simulink model "simulink_PD"  (R2024b)
settings: Solver=ode4  StartTime=0.0  StopTime=20  FixedStep=1e-3  RelTol=1e-3  EnableMultiTasking=on
values from neighbouring files (symbols this model uses):
  Kd = 100    [MAIN.m]
  Kp = 20000    [MAIN.m]
  noise = 0    [MAIN.m]
  V_ref = 60/3.6    (= 16.6666666667)    [MAIN.m]
undefined symbols (not defined in the file or in its folder): par
libraries: simulink x2
settings Model: Creator=bshyrokau  LastModifiedBy=nicvi
settings SolverCC: AlgebraicLoopSolver=TrustRegion
settings DataIOCC: SaveOutput=off  SignalLogging=off  DSMLogging=off  SaveTime=off  ReturnWorkspaceOutputs=off
settings OptimizationCC: ReuseModelBlockBuffer=off  LifeSpan=inf
settings DebuggingCC: UnconnectedInputMsg=warning  UnconnectedOutputMsg=warning  UnconnectedLineMsg=warning  AllowSymbolicDim=off  SFUnexpectedBacktrackingDiag=warning  SFNoUnconditionalDefaultTransitionDiag=warning  SFExecutionAtInitializationDiag=none  ArithmeticOperatorsInVariantConditions=warning
settings ModelReferenceCC: EnableRefExpFcnMdlSchedulingChecks=on  PropagateSignalLabelsOutOfModel=off
settings SFSimCC: SimUseLocalCustomCode=off  CustomCodeUndefinedFunction=UseInterfaceOnly
settings RTWCC: RTWUseLocalCustomCode=off  GPUComputeCapability=3.5  DLArmComputeVersion=19.05
settings CodeAppCC: StateflowObjectComments=on
settings GRTTargetCC: TargetLangStandard=C89/C90 (ANSI)
settings ConfigComp: CovMetricSettings=dw  CovSaveCumulativeToWorkspaceVar=on  CovSaveSingleToWorkspaceVar=on  CovExternalEMLEnable=off
settings SimscapeCC: SimscapeNormalizeSystem=off
settings ConfigurationSet: Description=SimMechanics 2G

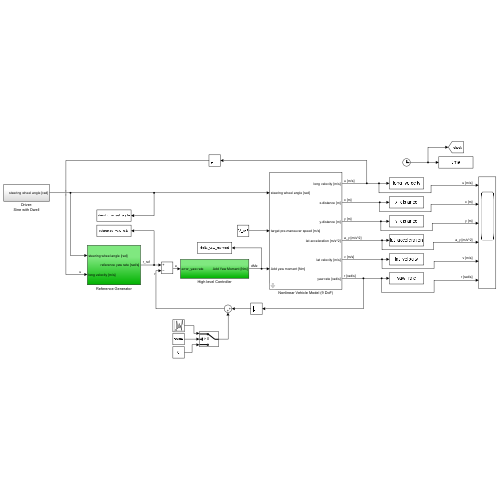
[thumbnail: Simulink's stored preview of the top-level diagram]
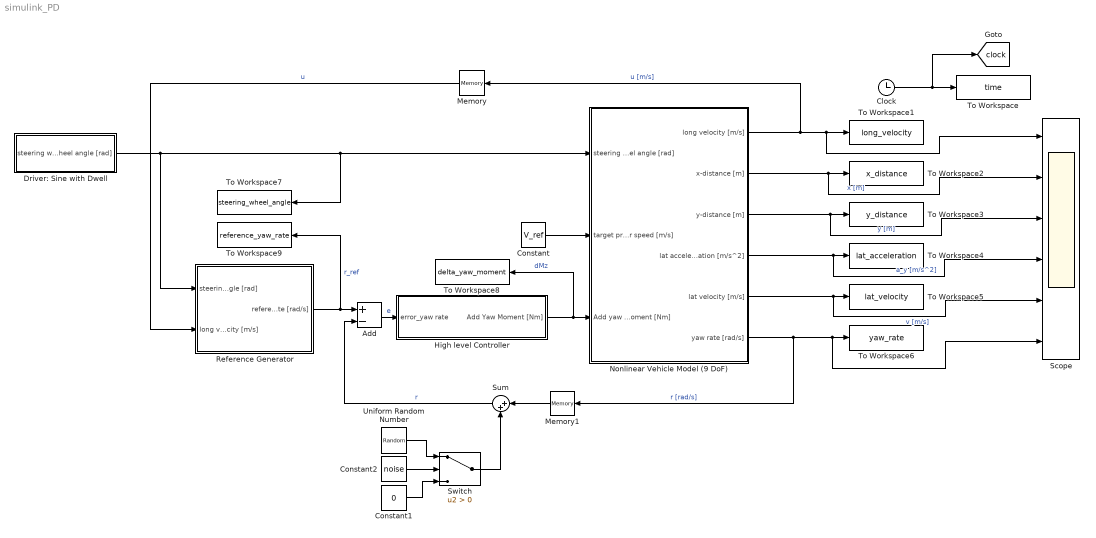
== system simulink_PD ==
  Add : Sum  Inputs=+-
  Clock : Clock
  Constant : Constant  Value=V_ref
  Constant1 : Constant  Value=0
  Constant2 : Constant  Value=noise
  Driver: Sine with Dwell : Subsystem
  High level Controller : Subsystem
  Memory : Memory
  Memory1 : Memory
  Nonlinear Vehicle Model (9 DoF) : Subsystem
      mask help: Simulink:masks:GenSFuncDesc_MD
      mask Help: eval('feval(''rtwprivate'',''rtwhelpview'',''rtw_sfcn_block'')');
  Reference Generator : Subsystem
  Scope : Scope  NumInputPorts=6
  Sum : Sum  Inputs=|++
  Switch : Switch  Criteria=u2 > Threshold  SaturateOnIntegerOverflow=off  InputSameDT=off
  To Workspace : ToWorkspace  VariableName=time  SampleTime=-1
  To Workspace1 : ToWorkspace  VariableName=long_velocity  SampleTime=-1
  To Workspace2 : ToWorkspace  VariableName=x_distance  SampleTime=-1
  To Workspace3 : ToWorkspace  VariableName=y_distance  SampleTime=-1
  To Workspace4 : ToWorkspace  VariableName=lat_acceleration  SampleTime=-1
  To Workspace5 : ToWorkspace  VariableName=lat_velocity  SampleTime=-1
  To Workspace6 : ToWorkspace  VariableName=yaw_rate  SampleTime=-1
  To Workspace7 : ToWorkspace  VariableName=steering_wheel_angle  SampleTime=-1
  To Workspace8 : ToWorkspace  VariableName=delta_yaw_moment  SampleTime=-1
  To Workspace9 : ToWorkspace  VariableName=reference_yaw_rate  SampleTime=-1
  Uniform Random Number : UniformRandomNumber  Minimum=-deg2rad(0.5)  Maximum=deg2rad(0.5)  SampleTime=0.001
  tag scope: clock=global
  wires:
  Driver: Sine with Dwell/1(steering wheel angle [rad]) -> Nonlinear Vehicle Model (9 DoF)/1(steering wheel angle [rad]), To Workspace7/1, Reference Generator/1(steering wheel angle [rad])
  Reference Generator/1(reference yaw rate [rad/s]) -> To Workspace9/1, Add/1  "r_ref"
  High level Controller/1(Add Yaw Moment [Nm]) -> To Workspace8/1, Nonlinear Vehicle Model (9 DoF)/3(Add yaw moment [Nm])  "dMz"
  Add/1 -> High level Controller/1(error_yaw rate)  "e"
  Nonlinear Vehicle Model (9 DoF)/6(yaw rate [rad/s]) -> Scope/6, To Workspace6/1, Memory1/1  "r [rad/s]"
  Nonlinear Vehicle Model (9 DoF)/5(lat velocity [m/s]) -> Scope/5, To Workspace5/1  "v [m/s]"
  Nonlinear Vehicle Model (9 DoF)/1(long velocity [m/s]) -> Scope/1, To Workspace1/1, Memory/1  "u [m/s]"
  Nonlinear Vehicle Model (9 DoF)/4(lat acceleration [m/s^2]) -> Scope/4, To Workspace4/1  "a_y [m/s^2]"
  Nonlinear Vehicle Model (9 DoF)/2(x-distance [m]) -> Scope/2, To Workspace2/1  "x [m]"
  Nonlinear Vehicle Model (9 DoF)/3(y-distance [m]) -> Scope/3, To Workspace3/1  "y [m]"
  Constant/1 -> Nonlinear Vehicle Model (9 DoF)/2(target pre-maneuver speed [m/s])
  Clock/1 -> [clock], To Workspace/1
  Memory/1 -> Reference Generator/2(long velocity [m/s])  "u"
  Memory1/1 -> Sum/1
  Uniform Random Number/1 -> Switch/1
  Sum/1 -> Add/2  "r"
  Switch/1 -> Sum/2
  Constant1/1 -> Switch/3
  Constant2/1 -> Switch/2

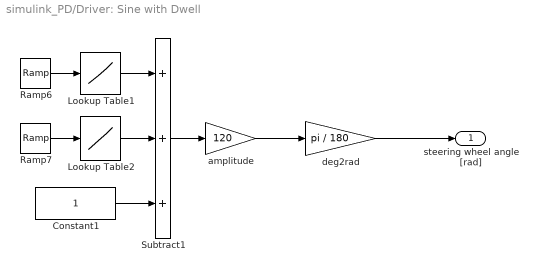
== system simulink_PD/Driver: Sine with Dwell ==
  Constant1 : Constant
  Lookup Table1 : Lookup  InputValues=[0:0.1:3*pi/2 3*pi/2+eps]*0.7  Table=sin([0:0.1:3*pi/2 3*pi/2+eps])  LookUpMeth=Interpolation-Use End Values  SaturateOnIntegerOverflow=off
  Lookup Table2 : Lookup  InputValues=[3*pi/2:0.1:2*pi 2*pi+eps]*0.7  Table=sin([3*pi/2:0.1:2*pi 2*pi+eps])  LookUpMeth=Interpolation-Use End Values  SaturateOnIntegerOverflow=off
  Ramp6 : simulink/Sources/Ramp  slope=pi  start=10  InitialOutput=0
  Ramp7 : simulink/Sources/Ramp  slope=pi  start=10+0.5  InitialOutput=0
  Subtract1 : Sum  Inputs=+++
  amplitude : Gain  Gain=120
  deg2rad : Gain  Gain=pi / 180
  steering wheel angle [rad] : Outport  VectorParamsAs1DForOutWhenUnconnected=off
  wires:
  Ramp6/1 -> Lookup Table1/1
  Ramp7/1 -> Lookup Table2/1
  Lookup Table2/1 -> Subtract1/2
  Lookup Table1/1 -> Subtract1/1
  Constant1/1 -> Subtract1/3
  Subtract1/1 -> amplitude/1
  amplitude/1 -> deg2rad/1
  deg2rad/1 -> steering wheel angle [rad]/1

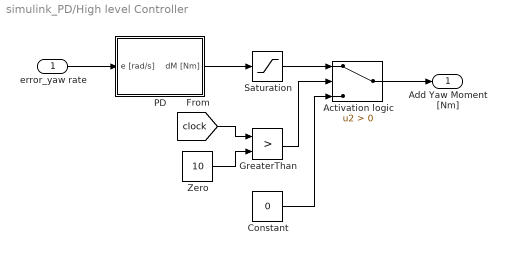
== system simulink_PD/High level Controller ==
  error_yaw rate : Inport
  Activation logic : Switch  Criteria=u2 > Threshold  SaturateOnIntegerOverflow=off  InputSameDT=off
  Constant : Constant  Value=0
  GreaterThan : RelationalOperator  Operator=>  OutDataTypeStr=boolean  RndMeth=Simplest  InputSameDT=off
  PD : Subsystem
  Saturation : Saturate  UpperLimit=10000  LowerLimit=-10000
  Zero : Constant  Value=10  OutDataTypeStr=Inherit: Inherit via back propagation
  Add Yaw Moment [Nm] : Outport  VectorParamsAs1DForOutWhenUnconnected=off
  wires:
  error_yaw rate/1 -> PD/1(e [rad/s])
  Saturation/1 -> Activation logic/1
  PD/1(dM [Nm]) -> Saturation/1
  Activation logic/1 -> Add Yaw Moment [Nm]/1
  Constant/1 -> Activation logic/3
  Zero/1 -> GreaterThan/2
  [clock] -> GreaterThan/1
  GreaterThan/1 -> Activation logic/2

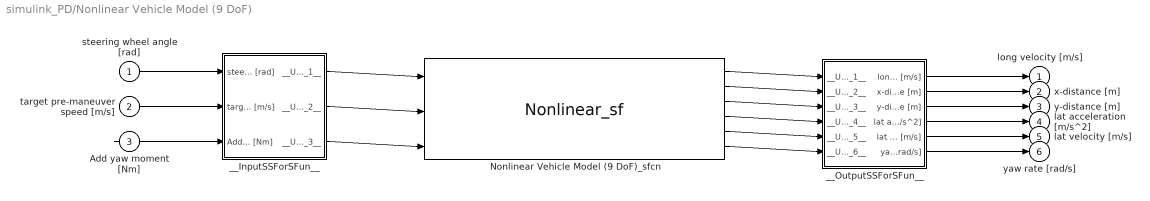
== system simulink_PD/Nonlinear Vehicle Model (9 DoF) ==
  steering wheel angle [rad] : Inport
  target pre-maneuver speed [m/s] : Inport  Port=2
  Add yaw moment [Nm] : Inport  Port=3
  Nonlinear Vehicle Model (9 DoF)_sfcn : S-Function  FunctionName=Nonlinear_sf  SFunctionModules=""  SFunctionDeploymentMode=off  EnableBusSupport=off  mask{rtw_sf_name=Nonlinear_sf, showVar=off}
      mask prompts: rtw_sf_name "Simulink:masks:GenSFuncName_MP"; showVar "Simulink:masks:GenSFuncShowModuleList_MP"
      mask help: Simulink:masks:GenSFuncDesc_MD
      mask init:
      | displist = '';
      | if ~strcmp(get_param(gcb, 'FunctionName'), rtw_sf_name);
      |   set_param(gcb, 'FunctionName', rtw_sf_name);
      | end
      | % Check if we are generating code
      | rtw_mode = false;
      | if strcmpi(get_param(bdroot(gcb),'SimulationStatus'),'Initializing')
      | 	rtw_mode = strcmpi(get_param(bdroot(gcb),'BuildingRTWCode'),'on') && ...
      | 		~strcmpi(get_param(bdroot(gcb),'TargetStyle'),'SimulationTarget');
      | end
      | if showVar || rtw_mode
      | 	if exist('rtwsfunc') == 2 | exist('rtwsfunc') == 6
      | 		tmplist = rtwsfunc(rtw_sf_name,gcb);
      | 		tmplist = DAStudio.message('Simulink:masks:GenSFuncListOfModules_IC', tmplist);
      | 	elseif showVar
      | 		tmplist1 = DAStudio.message('Simulink:masks:GenSFuncListOfModules_IC', '');
      |         tmplist2 = DAStudio.message('Simulink:masks:GenSFuncNotLicensed_IC');
      |         tmplist = [tmplist1 tmplist2];
      |  	end
      | end
      | if showVar
      |   displist = tmplist;
      | end
      settings: CopyFcn=|
      | if ~strcmp(get_param(gcb,'Linkstatus'),'none') && ...
      | ~strcmp(get_param(gcb,'Linkstatus'),'implicit')
      |   set_param(gcb,'LinkStatus','none');
      | end
      mask Help: eval('feval(''rtwprivate'',''rtwhelpview'',''rtw_sfcn_block'')');
      mask Display:
      | port_label('input',1,'steering wheel angle [rad]');
      | port_label('input',2,'target pre-maneuver speed [m/s]');
      | port_label('input',3,'Add yaw moment [Nm]');
      | port_label('output',1,'long velocity [m/s]');
      | port_label('output',2,'x-distance [m]');
      | port_label('output',3,'y-distance [m]');
      | port_label('output',4,'lat acceleration [m/s^2]');
      | port_label('output',5,'lat velocity [m/s]');
      | port_label('output',6,'yaw rate [rad/s]');
  __InputSSForSFun__ : Subsystem
  __OutputSSForSFun__ : Subsystem
  long velocity [m/s] : Outport  VectorParamsAs1DForOutWhenUnconnected=off
  x-distance [m] : Outport  Port=2  VectorParamsAs1DForOutWhenUnconnected=off
  y-distance [m] : Outport  Port=3  VectorParamsAs1DForOutWhenUnconnected=off
  lat acceleration [m/s^2] : Outport  Port=4  VectorParamsAs1DForOutWhenUnconnected=off
  lat velocity [m/s] : Outport  Port=5  VectorParamsAs1DForOutWhenUnconnected=off
  yaw rate [rad/s] : Outport  Port=6  VectorParamsAs1DForOutWhenUnconnected=off
  wires:
  steering wheel angle [rad]/1 -> __InputSSForSFun__/1(steering wheel angle [rad])
  target pre-maneuver speed [m/s]/1 -> __InputSSForSFun__/2(target pre-maneuver speed [m/s])
  Add yaw moment [Nm]/1 -> __InputSSForSFun__/3(Add yaw moment [Nm])
  __InputSSForSFun__/1(__UniqueOutportName__1__) -> Nonlinear Vehicle Model (9 DoF)_sfcn/1
  __InputSSForSFun__/2(__UniqueOutportName__2__) -> Nonlinear Vehicle Model (9 DoF)_sfcn/2
  __InputSSForSFun__/3(__UniqueOutportName__3__) -> Nonlinear Vehicle Model (9 DoF)_sfcn/3
  Nonlinear Vehicle Model (9 DoF)_sfcn/1 -> __OutputSSForSFun__/1(__UniqueInportName__1__)
  Nonlinear Vehicle Model (9 DoF)_sfcn/2 -> __OutputSSForSFun__/2(__UniqueInportName__2__)
  Nonlinear Vehicle Model (9 DoF)_sfcn/3 -> __OutputSSForSFun__/3(__UniqueInportName__3__)
  Nonlinear Vehicle Model (9 DoF)_sfcn/4 -> __OutputSSForSFun__/4(__UniqueInportName__4__)
  Nonlinear Vehicle Model (9 DoF)_sfcn/5 -> __OutputSSForSFun__/5(__UniqueInportName__5__)
  Nonlinear Vehicle Model (9 DoF)_sfcn/6 -> __OutputSSForSFun__/6(__UniqueInportName__6__)
  __OutputSSForSFun__/1(long velocity [m/s]) -> long velocity [m/s]/1
  __OutputSSForSFun__/2(x-distance [m]) -> x-distance [m]/1
  __OutputSSForSFun__/3(y-distance [m]) -> y-distance [m]/1
  __OutputSSForSFun__/4(lat acceleration [m/s^2]) -> lat acceleration [m/s^2]/1
  __OutputSSForSFun__/5(lat velocity [m/s]) -> lat velocity [m/s]/1
  __OutputSSForSFun__/6(yaw rate [rad/s]) -> yaw rate [rad/s]/1

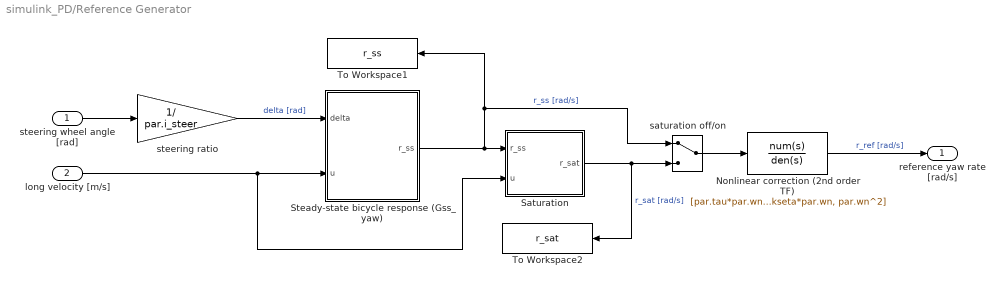
== system simulink_PD/Reference Generator ==
  steering wheel angle [rad] : Inport
  long velocity [m/s] : Inport  Port=2
  Nonlinear correction (2nd order TF) : TransferFcn  Numerator=[par.tau*par.wn^2, par.wn^2]  Denominator=[1, 2*par.kseta*par.wn, par.wn^2]
  Saturation : Subsystem
  Steady-state bicycle response (Gss_yaw) : Subsystem
  To Workspace1 : ToWorkspace  VariableName=r_ss  SampleTime=-1
  To Workspace2 : ToWorkspace  VariableName=r_sat  SampleTime=-1
  saturation off/on : ManualSwitch
  steering ratio : Gain  Gain=1/ par.i_steer
  reference yaw rate [rad/s] : Outport  VectorParamsAs1DForOutWhenUnconnected=off
  wires:
  steering wheel angle [rad]/1 -> steering ratio/1
  steering ratio/1 -> Steady-state bicycle response (Gss_yaw)/1(delta)  "delta [rad]"
  long velocity [m/s]/1 -> Saturation/2(u), Steady-state bicycle response (Gss_yaw)/2(u)
  Steady-state bicycle response (Gss_yaw)/1(r_ss) -> saturation off/on/1, To Workspace1/1, Saturation/1(r_ss)  "r_ss [rad/s]"
  Nonlinear correction (2nd order TF)/1 -> reference yaw rate [rad/s]/1  "r_ref [rad/s]"
  saturation off/on/1 -> Nonlinear correction (2nd order TF)/1
  Saturation/1(r_sat) -> To Workspace2/1, saturation off/on/2  "r_sat [rad/s]"

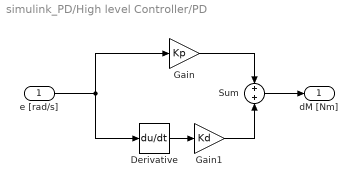
== system simulink_PD/High level Controller/PD ==
  e [rad/s] : Inport
  Derivative : Derivative
  Gain : Gain  Gain=Kp
  Gain1 : Gain  Gain=Kd
  Sum : Sum  Inputs=+|+
  dM [Nm] : Outport
  wires:
  Sum/1 -> dM [Nm]/1
  Gain1/1 -> Sum/2
  Gain/1 -> Sum/1
  e [rad/s]/1 -> Derivative/1, Gain/1
  Derivative/1 -> Gain1/1

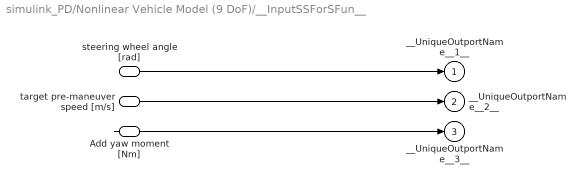
== system simulink_PD/Nonlinear Vehicle Model (9 DoF)/__InputSSForSFun__ ==
  steering wheel angle [rad] : Inport
  target pre-maneuver speed [m/s] : Inport  Port=2
  Add yaw moment [Nm] : Inport  Port=3
  __UniqueOutportName__1__ : Outport
  __UniqueOutportName__2__ : Outport  Port=2
  __UniqueOutportName__3__ : Outport  Port=3
  wires:
  steering wheel angle [rad]/1 -> __UniqueOutportName__1__/1
  target pre-maneuver speed [m/s]/1 -> __UniqueOutportName__2__/1
  Add yaw moment [Nm]/1 -> __UniqueOutportName__3__/1

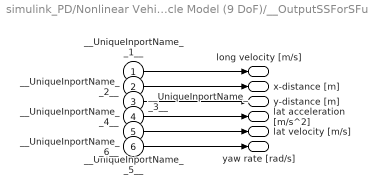
== system simulink_PD/Nonlinear Vehicle Model (9 DoF)/__OutputSSForSFun__ ==
  __UniqueInportName__1__ : Inport
  __UniqueInportName__2__ : Inport  Port=2
  __UniqueInportName__3__ : Inport  Port=3
  __UniqueInportName__4__ : Inport  Port=4
  __UniqueInportName__5__ : Inport  Port=5
  __UniqueInportName__6__ : Inport  Port=6
  long velocity [m/s] : Outport  VectorParamsAs1DForOutWhenUnconnected=off
  x-distance [m] : Outport  Port=2  VectorParamsAs1DForOutWhenUnconnected=off
  y-distance [m] : Outport  Port=3  VectorParamsAs1DForOutWhenUnconnected=off
  lat acceleration [m/s^2] : Outport  Port=4  VectorParamsAs1DForOutWhenUnconnected=off
  lat velocity [m/s] : Outport  Port=5  VectorParamsAs1DForOutWhenUnconnected=off
  yaw rate [rad/s] : Outport  Port=6  VectorParamsAs1DForOutWhenUnconnected=off
  wires:
  __UniqueInportName__1__/1 -> long velocity [m/s]/1
  __UniqueInportName__2__/1 -> x-distance [m]/1
  __UniqueInportName__3__/1 -> y-distance [m]/1
  __UniqueInportName__4__/1 -> lat acceleration [m/s^2]/1
  __UniqueInportName__5__/1 -> lat velocity [m/s]/1
  __UniqueInportName__6__/1 -> yaw rate [rad/s]/1

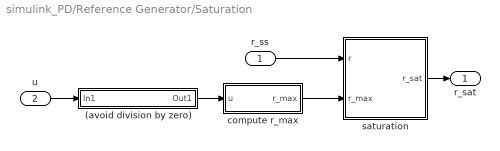
== system simulink_PD/Reference Generator/Saturation ==
  r_ss : Inport
  u : Inport  Port=2
  (avoid division by zero) : Subsystem
  compute r_max : Subsystem
  saturation : MATLAB Function  TreatAsAtomicUnit=on
  r_sat : Outport
  wires:
  compute r_max/1(r_max) -> saturation/2(r_max)
  saturation/1(r_sat) -> r_sat/1
  r_ss/1 -> saturation/1(r)
  u/1 -> (avoid division by zero)/1(In1)
  (avoid division by zero)/1(Out1) -> compute r_max/1(u)

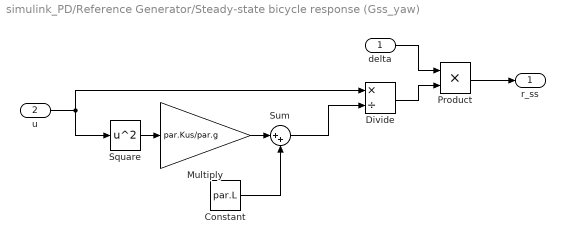
== system simulink_PD/Reference Generator/Steady-state bicycle response (Gss_yaw) ==
  delta : Inport
  u : Inport  Port=2
  Constant : Constant  Value=par.L
  Divide : Product  Inputs=*/
  Multiply : Gain  Gain=par.Kus/par.g
  Product : Product
  Square : Math  Operator=square
  Sum : Sum  Inputs=|++
  r_ss : Outport
  wires:
  u/1 -> Square/1, Divide/1
  Square/1 -> Multiply/1
  Multiply/1 -> Sum/1
  Constant/1 -> Sum/2
  Sum/1 -> Divide/2
  delta/1 -> Product/1
  Divide/1 -> Product/2
  Product/1 -> r_ss/1

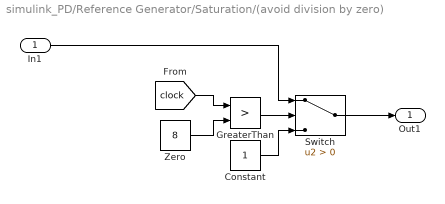
== system simulink_PD/Reference Generator/Saturation/(avoid division by zero) ==
  In1 : Inport
  Constant : Constant
  GreaterThan : RelationalOperator  Operator=>  OutDataTypeStr=boolean  RndMeth=Simplest  InputSameDT=off
  Switch : Switch  Criteria=u2 > Threshold  SaturateOnIntegerOverflow=off  InputSameDT=off
  Zero : Constant  Value=8  OutDataTypeStr=Inherit: Inherit via back propagation
  Out1 : Outport
  wires:
  Constant/1 -> Switch/3
  [clock] -> GreaterThan/1
  GreaterThan/1 -> Switch/2
  Switch/1 -> Out1/1
  In1/1 -> Switch/1
  Zero/1 -> GreaterThan/2

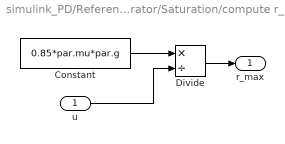
== system simulink_PD/Reference Generator/Saturation/compute r_max ==
  u : Inport
  Constant : Constant  Value=0.85*par.mu*par.g
  Divide : Product  Inputs=*/
  r_max : Outport
  wires:
  Constant/1 -> Divide/1
  Divide/1 -> r_max/1
  u/1 -> Divide/2

== matlab function simulink_PD/Reference Generator/Saturation/saturation ==
  data: r input; r_sat output; r_max input
function r_sat=sat(r,r_max)

if r>r_max
    r_sat=r_max;
elseif r<-r_max
    r_sat=-r_max;
else
    r_sat=r;
end

end
